simulink model "TB3_Formation_Simulation"  (R2019b)
settings: Solver=VariableStepAuto  StartTime=0.0  StopTime=10.0  RelTol=1e-3
values from neighbouring files (symbols this model uses):
  Adj_VL = [Adj connect; connect' 0]    [graph_create.m]
  Kp_alpha = 15    [main.m]
  Kp_beta = -6    [main.m]
  Kp_rho = 9    [main.m]
  N = 6    [main.m]
  r_rel_1 = r_rel_ploy    [create_r_relative.m]
undefined symbols (not defined in the file or in its folder): DiscIntNeverNeededParam
libraries: mobileRoboticsLib x3
settings Model: Creator=chant  LastModifiedBy=chant

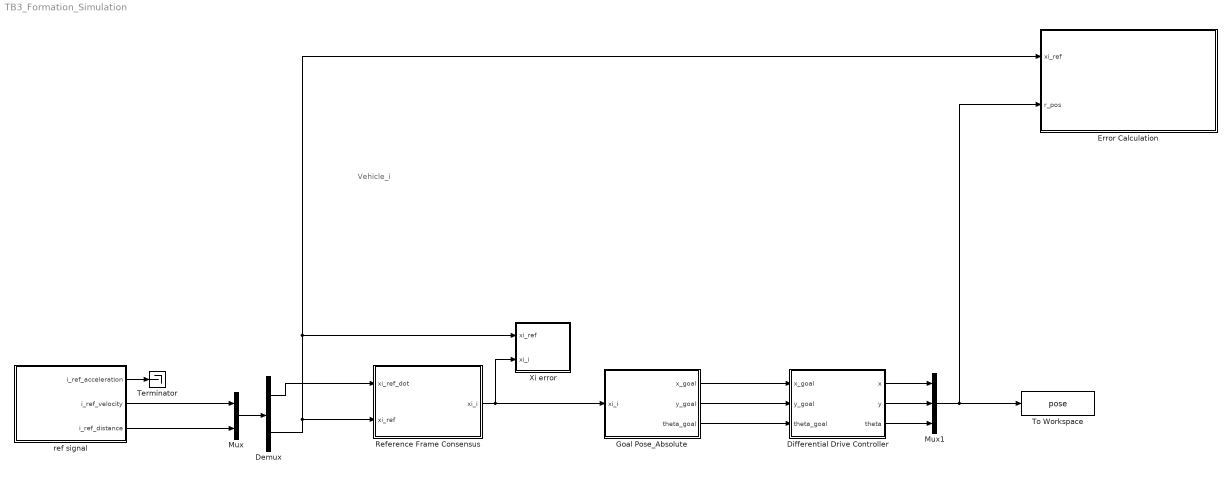
== system TB3_Formation_Simulation ==
  note: Vehicle_i
  Demux : Demux  Outputs=2
  Differential Drive Controller : Subsystem
  Error Calculation : Subsystem
  Goal Pose_Absolute : Subsystem
  Mux : Mux  Inputs=2
  Mux1 : Mux  Inputs=3
  Reference Frame Consensus : Subsystem
  Terminator : Terminator
  To Workspace : ToWorkspace  VariableName=pose  SaveFormat=Timeseries  SampleTime=-1
  Xi error : Subsystem
  ref signal : Subsystem
  wires:
  Reference Frame Consensus/1(xi_i) -> Xi error/2(xi_i), Goal Pose_Absolute/1(xi_i)
  Goal Pose_Absolute/1(x_goal) -> Differential Drive Controller/1(x_goal)
  Goal Pose_Absolute/2(y_goal) -> Differential Drive Controller/2(y_goal)
  Goal Pose_Absolute/3(theta_goal) -> Differential Drive Controller/3(theta_goal)
  Demux/2 -> Error Calculation/1(xi_ref), Xi error/1(xi_ref), Reference Frame Consensus/2(xi_ref)
  ref signal/2(i_ref_velocity) -> Mux/1
  ref signal/3(i_ref_distance) -> Mux/2
  Mux/1 -> Demux/1
  Demux/1 -> Reference Frame Consensus/1(xi_ref_dot)
  Differential Drive Controller/1(x) -> Mux1/1
  Differential Drive Controller/2(y) -> Mux1/2
  Differential Drive Controller/3(theta) -> Mux1/3
  Mux1/1 -> Error Calculation/2(r_pos), To Workspace/1
  ref signal/1(i_ref_acceleration) -> Terminator/1

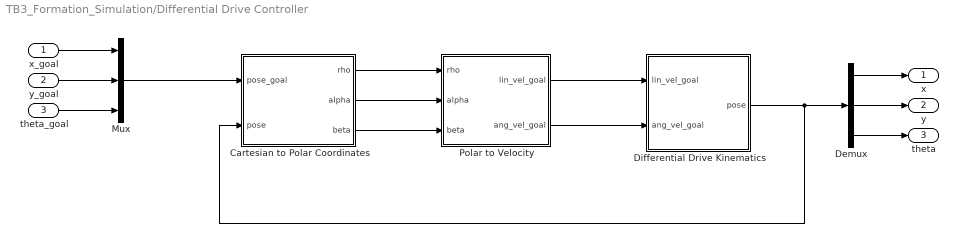
== system TB3_Formation_Simulation/Differential Drive Controller ==
  x_goal : Inport
  y_goal : Inport  Port=2
  theta_goal : Inport  Port=3
  Cartesian to Polar Coordinates : MATLAB Function  TreatAsAtomicUnit=on
  Demux : Demux  Outputs=3
  Differential Drive Kinematics : Subsystem
  Mux : Mux  Inputs=3
  Polar to Velocity : Subsystem
  x : Outport
  y : Outport  Port=2
  theta : Outport  Port=3
  wires:
  Differential Drive Kinematics/1(pose) -> Demux/1, Cartesian to Polar Coordinates/2(pose)
  Demux/1 -> x/1
  Demux/3 -> theta/1
  Demux/2 -> y/1
  Mux/1 -> Cartesian to Polar Coordinates/1(pose_goal)
  theta_goal/1 -> Mux/3
  y_goal/1 -> Mux/2
  x_goal/1 -> Mux/1
  Cartesian to Polar Coordinates/2(alpha) -> Polar to Velocity/2(alpha)
  Cartesian to Polar Coordinates/1(rho) -> Polar to Velocity/1(rho)
  Cartesian to Polar Coordinates/3(beta) -> Polar to Velocity/3(beta)
  Polar to Velocity/1(lin_vel_goal) -> Differential Drive Kinematics/1(lin_vel_goal)
  Polar to Velocity/2(ang_vel_goal) -> Differential Drive Kinematics/2(ang_vel_goal)

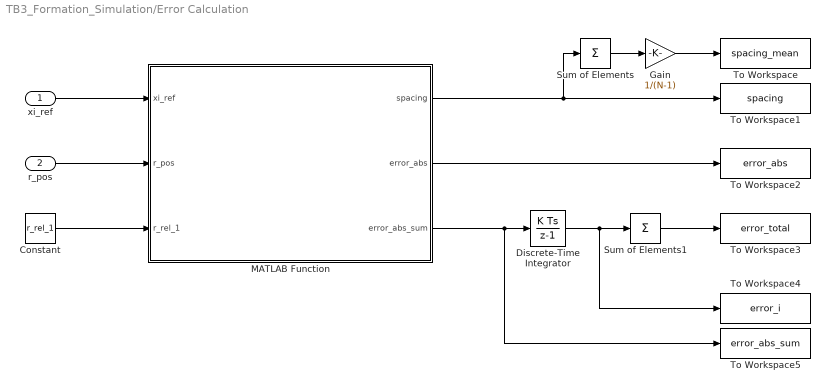
== system TB3_Formation_Simulation/Error Calculation ==
  xi_ref : Inport
  r_pos : Inport  Port=2
  Constant : Constant  Value=r_rel_1
  Discrete-Time Integrator : DiscreteIntegrator  SampleTime=-1  ICPrevOutput=DiscIntNeverNeededParam  ICPrevScaledInput=DiscIntNeverNeededParam
  Gain : Gain  Gain=1/(N-1)
  MATLAB Function : MATLAB Function  TreatAsAtomicUnit=on
  Sum of Elements : Sum  Inputs=+
  Sum of Elements1 : Sum  Inputs=+
  To Workspace : ToWorkspace  VariableName=spacing_mean  SaveFormat=Timeseries  SampleTime=-1
  To Workspace1 : ToWorkspace  VariableName=spacing  SaveFormat=Timeseries  SampleTime=-1
  To Workspace2 : ToWorkspace  VariableName=error_abs  SaveFormat=Timeseries  SampleTime=-1
  To Workspace3 : ToWorkspace  VariableName=error_total  SaveFormat=Timeseries  SampleTime=-1
  To Workspace4 : ToWorkspace  VariableName=error_i  SaveFormat=Timeseries  SampleTime=-1
  To Workspace5 : ToWorkspace  VariableName=error_abs_sum  SaveFormat=Timeseries  SampleTime=-1
  wires:
  Sum of Elements/1 -> Gain/1
  MATLAB Function/3(error_abs_sum) -> Discrete-Time Integrator/1, To Workspace5/1
  Constant/1 -> MATLAB Function/3(r_rel_1)
  MATLAB Function/2(error_abs) -> To Workspace2/1
  xi_ref/1 -> MATLAB Function/1(xi_ref)
  Sum of Elements1/1 -> To Workspace3/1
  Discrete-Time Integrator/1 -> To Workspace4/1, Sum of Elements1/1
  Gain/1 -> To Workspace/1
  MATLAB Function/1(spacing) -> To Workspace1/1, Sum of Elements/1
  r_pos/1 -> MATLAB Function/2(r_pos)

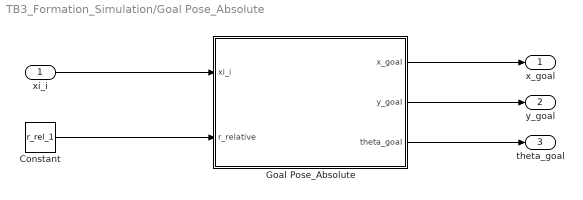
== system TB3_Formation_Simulation/Goal Pose_Absolute ==
  xi_i : Inport
  Constant : Constant  Value=r_rel_1
  Goal Pose_Absolute : MATLAB Function  TreatAsAtomicUnit=on
  x_goal : Outport
  y_goal : Outport  Port=2
  theta_goal : Outport  Port=3
  wires:
  xi_i/1 -> Goal Pose_Absolute/1(xi_i)
  Constant/1 -> Goal Pose_Absolute/2(r_relative)
  Goal Pose_Absolute/1(x_goal) -> x_goal/1
  Goal Pose_Absolute/2(y_goal) -> y_goal/1
  Goal Pose_Absolute/3(theta_goal) -> theta_goal/1

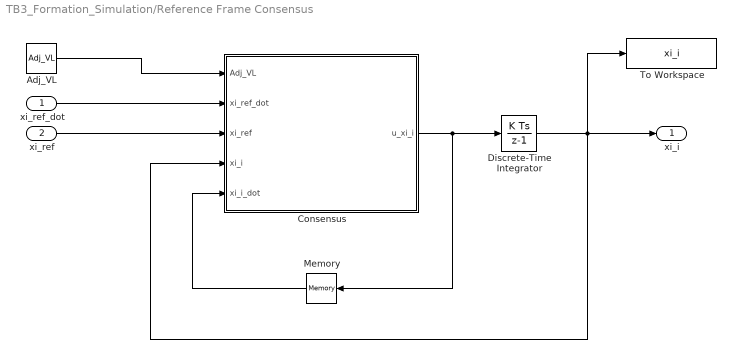
== system TB3_Formation_Simulation/Reference Frame Consensus ==
  xi_ref_dot : Inport
  xi_ref : Inport  Port=2
  Adj_VL : Constant  Value=Adj_VL
  Consensus : MATLAB Function  TreatAsAtomicUnit=on
  Discrete-Time Integrator : DiscreteIntegrator  SampleTime=-1  ICPrevOutput=DiscIntNeverNeededParam  ICPrevScaledInput=DiscIntNeverNeededParam
  Memory : Memory
  To Workspace : ToWorkspace  VariableName=xi_i  SaveFormat=Timeseries  SampleTime=-1
  xi_i : Outport
  wires:
  Adj_VL/1 -> Consensus/1(Adj_VL)
  xi_ref_dot/1 -> Consensus/2(xi_ref_dot)
  xi_ref/1 -> Consensus/3(xi_ref)
  Consensus/1(u_xi_i) -> Discrete-Time Integrator/1, Memory/1
  Memory/1 -> Consensus/5(xi_i_dot)
  Discrete-Time Integrator/1 -> Consensus/4(xi_i), To Workspace/1, xi_i/1

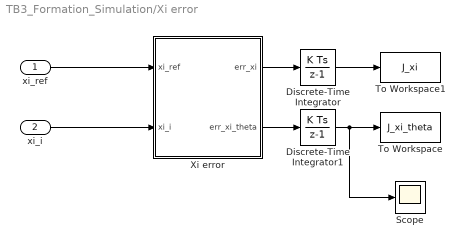
== system TB3_Formation_Simulation/Xi error ==
  xi_ref : Inport
  xi_i : Inport  Port=2
  Discrete-Time Integrator : DiscreteIntegrator  SampleTime=-1  ICPrevOutput=DiscIntNeverNeededParam  ICPrevScaledInput=DiscIntNeverNeededParam
  Discrete-Time Integrator1 : DiscreteIntegrator  SampleTime=-1  ICPrevOutput=DiscIntNeverNeededParam  ICPrevScaledInput=DiscIntNeverNeededParam
  Scope : Scope
  To Workspace : ToWorkspace  VariableName=J_xi_theta  SaveFormat=Timeseries  SampleTime=-1
  To Workspace1 : ToWorkspace  VariableName=J_xi  SaveFormat=Timeseries  SampleTime=-1
  Xi error : MATLAB Function  TreatAsAtomicUnit=on
  wires:
  Xi error/1(err_xi) -> Discrete-Time Integrator/1
  Discrete-Time Integrator/1 -> To Workspace1/1
  xi_ref/1 -> Xi error/1(xi_ref)
  xi_i/1 -> Xi error/2(xi_i)
  Xi error/2(err_xi_theta) -> Discrete-Time Integrator1/1
  Discrete-Time Integrator1/1 -> Scope/1, To Workspace/1

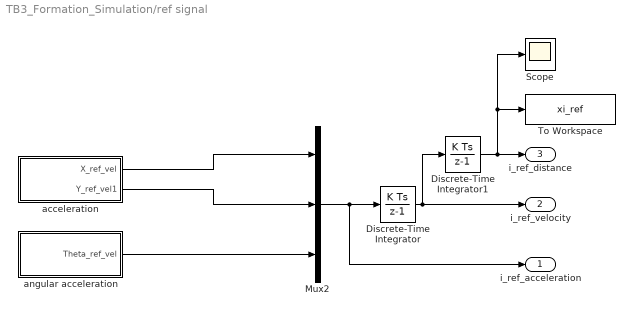
== system TB3_Formation_Simulation/ref signal ==
  Discrete-Time Integrator : DiscreteIntegrator  SampleTime=-1  ICPrevOutput=DiscIntNeverNeededParam  ICPrevScaledInput=DiscIntNeverNeededParam
  Discrete-Time Integrator1 : DiscreteIntegrator  SampleTime=-1  ICPrevOutput=DiscIntNeverNeededParam  ICPrevScaledInput=DiscIntNeverNeededParam
  Mux2 : Mux  Inputs=3
  Scope : Scope
  To Workspace : ToWorkspace  VariableName=xi_ref  SaveFormat=Timeseries  SampleTime=-1
  acceleration : Subsystem  TreatAsAtomicUnit=on
  angular acceleration : Subsystem  TreatAsAtomicUnit=on
  i_ref_acceleration : Outport
  i_ref_velocity : Outport  Port=2
  i_ref_distance : Outport  Port=3
  wires:
  acceleration/1(X_ref_vel) -> Mux2/1
  angular acceleration/1(Theta_ref_vel) -> Mux2/3
  acceleration/2(Y_ref_vel1) -> Mux2/2
  Mux2/1 -> Discrete-Time Integrator/1, i_ref_acceleration/1
  Discrete-Time Integrator/1 -> i_ref_velocity/1, Discrete-Time Integrator1/1
  Discrete-Time Integrator1/1 -> To Workspace/1, Scope/1, i_ref_distance/1

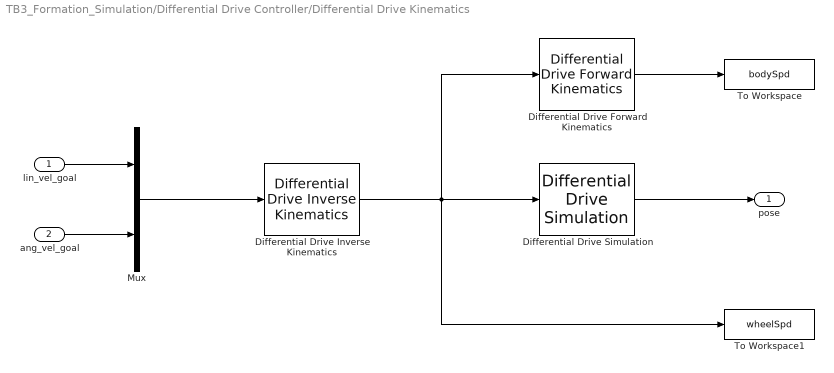
== system TB3_Formation_Simulation/Differential Drive Controller/Differential Drive Kinematics ==
  lin_vel_goal : Inport
  ang_vel_goal : Inport  Port=2
  Differential Drive Forward Kinematics : mobileRoboticsLib/Kinematic Models/Differential Drive/Differential Drive Forward Kinematics  wheelRadius=0.033  wheelBase=0.16
      settings: SourceProductName=Mobile Robotics Simulation Toolbox
  Differential Drive Inverse Kinematics : mobileRoboticsLib/Kinematic Models/Differential Drive/Differential Drive Inverse Kinematics  wheelRadius=0.033  wheelBase=0.16
      settings: SourceProductName=Mobile Robotics Simulation Toolbox
  Differential Drive Simulation : mobileRoboticsLib/Kinematic Models/Differential Drive/Differential Drive Simulation  wheelRadius=0.033  wheelBase=0.16  initX=0  initY=0  initAngle=0  Ts=0.01
      settings: SourceProductName=Mobile Robotics Simulation Toolbox
  Mux : Mux  Inputs=2
  To Workspace : ToWorkspace  VariableName=bodySpd  SaveFormat=Timeseries  SampleTime=-1
  To Workspace1 : ToWorkspace  VariableName=wheelSpd  SaveFormat=Timeseries  SampleTime=-1
  pose : Outport
  wires:
  Differential Drive Inverse Kinematics/1 -> To Workspace1/1, Differential Drive Forward Kinematics/1, Differential Drive Simulation/1
  lin_vel_goal/1 -> Mux/1
  ang_vel_goal/1 -> Mux/2
  Mux/1 -> Differential Drive Inverse Kinematics/1
  Differential Drive Forward Kinematics/1 -> To Workspace/1
  Differential Drive Simulation/1 -> pose/1

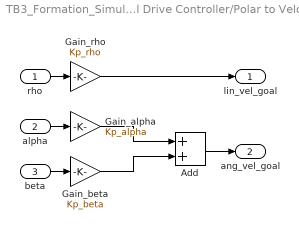
== system TB3_Formation_Simulation/Differential Drive Controller/Polar to Velocity ==
  rho : Inport
  alpha : Inport  Port=2
  beta : Inport  Port=3
  Add : Sum
  Gain_alpha : Gain  Gain=Kp_alpha
  Gain_beta : Gain  Gain=Kp_beta
  "Gain_rho " : Gain  Gain=Kp_rho
  lin_vel_goal : Outport
  ang_vel_goal : Outport  Port=2
  wires:
  rho/1 -> "Gain_rho "/1
  Gain_alpha/1 -> Add/1
  "Gain_rho "/1 -> lin_vel_goal/1
  Gain_beta/1 -> Add/2
  beta/1 -> Gain_beta/1
  Add/1 -> ang_vel_goal/1
  alpha/1 -> Gain_alpha/1

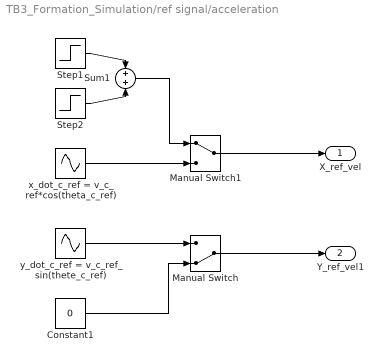
== system TB3_Formation_Simulation/ref signal/acceleration ==
  Constant1 : Constant  Value=0
  Manual Switch : ManualSwitch  CurrentSetting=0
  Manual Switch1 : ManualSwitch
  Step1 : Step  Time=0  After=0.4  SampleTime=0
  Step2 : Step  Time=2  After=-0.4  SampleTime=0
  Sum1 : Sum
  x_dot_c_ref = v_c_ref*cos(theta_c_ref) : Sin  Amplitude=9*pi/500  Frequency=pi/50  Phase=pi/2  SampleTime=0
  y_dot_c_ref = v_c_ref_sin(thete_c_ref) : Sin  Amplitude=9*pi/500  Frequency=pi/50  SampleTime=0
  X_ref_vel : Outport
  Y_ref_vel1 : Outport  Port=2
  wires:
  Manual Switch1/1 -> X_ref_vel/1
  Step1/1 -> Sum1/1
  Step2/1 -> Sum1/2
  y_dot_c_ref = v_c_ref_sin(thete_c_ref)/1 -> Manual Switch/1
  Manual Switch/1 -> Y_ref_vel1/1
  Constant1/1 -> Manual Switch/2
  Sum1/1 -> Manual Switch1/1
  x_dot_c_ref = v_c_ref*cos(theta_c_ref)/1 -> Manual Switch1/2

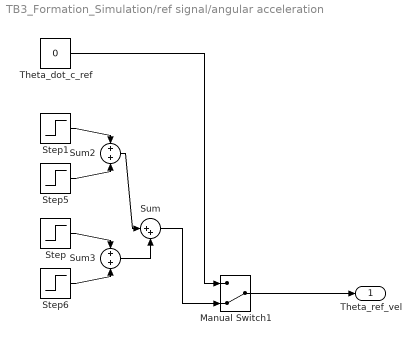
== system TB3_Formation_Simulation/ref signal/angular acceleration ==
  Manual Switch1 : ManualSwitch  CurrentSetting=0
  Step : Step  Time=5  After=-pi/2  SampleTime=0
  Step1 : Step  Time=4  After=pi/2  SampleTime=0
  Step5 : Step  Time=5  After=-pi/2  SampleTime=0
  Step6 : Step  Time=6  After=pi/2  SampleTime=0
  Sum : Sum  Inputs=|++
  Sum2 : Sum
  Sum3 : Sum
  Theta_dot_c_ref : Constant  Value=0
  Theta_ref_vel : Outport
  wires:
  Step/1 -> Sum3/1
  Step6/1 -> Sum3/2
  Theta_dot_c_ref/1 -> Manual Switch1/1
  Manual Switch1/1 -> Theta_ref_vel/1
  Sum3/1 -> Sum/2
  Sum/1 -> Manual Switch1/2
  Step5/1 -> Sum2/2
  Step1/1 -> Sum2/1
  Sum2/1 -> Sum/1

== matlab function TB3_Formation_Simulation/Reference Frame Consensus/Consensus ==
  data: Adj_VL input; u_xi_i output; xi_ref_dot input; xi_ref input; xi_i input; xi_i_dot input
function u_xi_i = consensus_xi(Adj_VL, xi_ref_dot, xi_ref, xi_i, xi_i_dot)
%CONSENSUS_XI calculates u_xi = xi_i_dot for all vehicles according to the consensus
%formula for time-varying reference state (access to the leader only to a subgroup)
% Inputs:
%       Adj_VL      - adjacency matrix
%       xi_ref_dot  - time derivative of the reference xi
%       xi_ref      - reference xi
%       xi_i        - vehicle i own understanding of reference frame
%       xi_i_dot    - vehicles i own understanding of the time derivative of xi
% Outputs:
%       u_xi_i       - control input of the i-th reference frame

% Number of vehicles
N = size(Adj_VL,1) - 1;
% initialize output u_xi to zero
u_xi_i = zeros(3,N);

% scalar to influence convergence speed
gamma = 1;

% formula to calculate xi_dot_i = u_i for each vehicle compare to thesis
% u consists of six states per vehicle in a 6xN matrix / updates each
% vehicle after another (6 states per iteration of outer for loop)
for i=1:1:N
    eta = sum(Adj_VL(i,:));
    % if vehicle has no incoming connection (equal to eta = 0) u is set to zero therefore the
    % information states don't change and remain constant
    if (eta == 0)
        u_xi_i(:,i) = zeros(3,1);
    else
        temp = zeros(3,1);
        for j=1:1:N
            temp = temp + Adj_VL(i,j)*(xi_i_dot(:,j) - gamma*(xi_i(:,i) - xi_i(:,j)));
        end
        u_xi_i(:,i) = 1/eta * temp + 1/eta * Adj_VL(i,N+1)*(xi_ref_dot-gamma*(xi_i(:,i)-xi_ref));
    end    
end

== matlab function TB3_Formation_Simulation/Error Calculation/MATLAB Function ==
  data: xi_ref input; spacing output; r_pos input; r_rel_1 input; error_abs output; error_abs_sum output
function [spacing,error_abs,error_abs_sum] = err_calc(xi_ref, r_pos, r_rel_1)
%ERR_CALC calculates the squared error between the given reference frame
%xi_ref and each vehicle actual position.
%
% Input:
%     xi_ref       - virtual reference frame (x,y,theta)
%     r_pos        - position vector of vehicles
%     r_rel        - relative positions of vehicles in formation
% Output:
%     err_total    - total squared errror over all vehicles
%     err_i        - individual error per vehicle
%     err_coord    - error per coordinate axis
%     

% number of vehicles
N = size(r_pos,2);

% calculate desired absolute positions based on xi_ref
r_des_abs = zeros(size(r_pos));

theta = xi_ref(3);

% rotational matrix
Dz = [cos(theta) -sin(theta) 0
      sin(theta)  cos(theta) 0
      0           0          1];

%loop over each vehicle
for i=1:1:N     
    r_des_abs(:,i) = xi_ref(:) + Dz*r_rel_1(:,i);    
end

error = r_pos - r_des_abs;
error_abs = abs(error); 
error_abs_sum = sum(error_abs(1:2,:),1);
%squared error

%distance between vehicles
veh_spacing = sqrt(sum(diff(r_pos').^2,2));
veh_spacing_should = ones(N-1,1)*0.8;

spacing = abs(veh_spacing);

== matlab function TB3_Formation_Simulation/Goal Pose_Absolute/Goal Pose_Absolute ==
  data: xi_i input; x_goal output; r_relative input; y_goal output; theta_goal output
function [x_goal,y_goal,theta_goal]  = goal_pose_abs(xi_i, r_relative)
%DESIRED_POS_ABS computes the desired absolute positions depending on the
%reference frame of the vehicle and the relative coordinates of the desired
%formation (three dimensional coordinate transformation)
%
% Inputs:
%       xi_i    - reference frame of the i-th vehicle
%       r_relative  - vehicle formation shape in the reference frame
% Outputs:
%       x_goal       - goal x-position of the vehicle
%       y_goal       - goal y-position of the vehicle
%       theta_goal   - goal theta-orientation of the vehicle

% set matrix nxn
% r_des  - combination of x,y,z-position in a matrix for all vehicles
r_des = zeros(size(r_relative));

%loop over each vehicle
for i=1:1:size(r_relative,2)
    
    % information state of the vehicle angle
    theta = xi_i(3,i);
    
    % rotational matrix
    Dz = [cos(theta) -sin(theta) 0
          sin(theta)  cos(theta) 0
          0           0          1];
     
    r_des(:,i) = xi_i(1:3,i) + Dz*r_relative(:,i);
end

x_goal = r_des(1,:);
y_goal = r_des(2,:);
theta_goal = r_des(3,:);

end

== matlab function TB3_Formation_Simulation/Differential Drive Controller/Cartesian to Polar Coordinates ==
  data: pose_goal input; rho output; pose input; alpha output; beta output
function [rho, alpha, beta] = Carte_to_Polar(pose_goal, pose)
% **Description:
% This function convert the current pose and goal pose information to rho,
% alpha and beta for each robot agent
%
% **Variables Description:
%   Inputs:
%       pose_goal   - goal pose
%       pose:       - current pose
%
%   Outputs:
%       rho         - Euclidean distance between the current pose and Goal pose
%       alpha       - Difference between goal and current orientation (angle)
%       beta        - Goal orientation (angle)

x_goal = pose_goal(1);
y_goal = pose_goal(2);

x = pose(1);
y = pose(2);
theta = pose(3);

% Convert Parameters:
x_delta = x_goal - x;
y_delta = y_goal - y;

% Output:
rho    = sqrt(x_delta.^2 + y_delta.^2);
alpha  = atan(y_delta/x_delta) - theta;
beta   = - theta - alpha;

== matlab function TB3_Formation_Simulation/Xi error/Xi error ==
  data: xi_ref input; err_xi output; xi_i input; err_xi_theta output
function [err_xi, err_xi_theta] = err_ref(xi_ref, xi_i)
%ERR_REF computes the error between the vehicles information state and
%reference information.
% 
% Input:
%       - xi_ref    reference information state
%       - xi_i      vehicle information state
% Output:
%       - err_xi    absolute xi error

err_xi = abs(xi_ref*ones(1,size(xi_i,2)) - xi_i);
err_xi_theta = err_xi(3,:);
